simulink model "DrivetrainEv"  (R2023a)
settings: Solver=VariableStepAuto  StartTime=0.0  StopTime=inf  RelTol=1e-3  EnableMultiTasking=on
model workspace (MAT data in the model file):
  Af = Simulink.Parameter
  Af.Value = 2.27
  Af.DataType = 'double'
  Af.Complexity = 'real'
  Af.Dimensions = [1 1]
  Bx = Simulink.Parameter
  Bx.Value = 10
  Bx.DataType = 'double'
  Bx.Complexity = 'real'
  Bx.Dimensions = [1 1]
  Cd = Simulink.Parameter
  Cd.Value = 0.28
  Cd.DataType = 'double'
  Cd.Complexity = 'real'
  Cd.Dimensions = [1 1]
  Cl = Simulink.Parameter
  Cl.Value = 0.1
  Cl.DataType = 'double'
  Cl.Complexity = 'real'
  Cl.Dimensions = [1 1]
  Cpm = Simulink.Parameter
  Cpm.Value = 0.1
  Cpm.DataType = 'double'
  Cpm.Complexity = 'real'
  Cpm.Dimensions = [1 1]
  Cx = Simulink.Parameter
  Cx.Value = 1.65
  Cx.DataType = 'double'
  Cx.Complexity = 'real'
  Cx.Dimensions = [1 1]
  Dx = Simulink.Parameter
  Dx.Value = 1
  Dx.DataType = 'double'
  Dx.Complexity = 'real'
  Dx.Dimensions = [1 1]
  Ex = Simulink.Parameter
  Ex.Value = 0.01
  Ex.DataType = 'double'
  Ex.Complexity = 'real'
  Ex.Dimensions = [1 1]
  FZMAX = Simulink.Parameter
  FZMAX.Value = 6570
  FZMAX.DataType = 'double'
  FZMAX.Complexity = 'real'
  FZMAX.Dimensions = [1 1]
  FZMIN = Simulink.Parameter
  FZMIN.Value = 0
  FZMIN.DataType = 'double'
  FZMIN.Complexity = 'real'
  FZMIN.Dimensions = [1 1]
  Fc = Simulink.Parameter
  Fc.Value = 500
  Fc.DataType = 'double'
  Fc.Complexity = 'real'
  Fc.Dimensions = [1 1]
  FsbF = Simulink.Parameter
  FsbF.Value = [-700000 -7000 -700 0 700 7000 700000]
  FsbF.DataType = 'double'
  FsbF.Complexity = 'real'
  FsbF.Dimensions = [1 7]
  FsbR = Simulink.Parameter
  FsbR.Value = [-700000 -7000 -700 0 700 7000 700000]
  FsbR.DataType = 'double'
  FsbR.Complexity = 'real'
  FsbR.Dimensions = [1 7]
  FskF = Simulink.Parameter
  FskF.Value = [-8928.57142857 -178.571428571 0 357.142857143 535.714285714 9285.71428571]
  FskF.DataType = 'double'
  FskF.Complexity = 'real'
  FskF.Dimensions = [1 6]
  FskR = Simulink.Parameter
  FskR.Value = [-5357.14285714 -107.142857143 0 214.285714286 321.428571429 5571.42857143]
  FskR.DataType = 'double'
  FskR.Complexity = 'real'
  FskR.Dimensions = [1 6]
  Iyy = Simulink.Parameter
  Iyy.Value = 3000
  Iyy.DataType = 'double'
  Iyy.Complexity = 'real'
  Iyy.Dimensions = [1 1]
  Iyy_Whl = Simulink.Parameter
  Iyy_Whl.Value = 0.8
  Iyy_Whl.DataType = 'double'
  Iyy_Whl.Complexity = 'real'
  Iyy_Whl.Dimensions = [1 1]
  J = Simulink.Parameter
  J.Value = 0.01
  J.DataType = 'double'
  J.Complexity = 'real'
  J.Dimensions = [1 1]
  Jd = Simulink.Parameter
  Jd.Value = 0.025
  Jd.DataType = 'double'
  Jd.Complexity = 'real'
  Jd.Dimensions = [1 1]
  Jmotor = Simulink.Parameter
  Jmotor.Value = 0.1
  Jmotor.DataType = 'double'
  Jmotor.Complexity = 'real'
  Jmotor.Dimensions = [1 1]
  Jw1 = Simulink.Parameter
  Jw1.Value = 0.01
  Jw1.DataType = 'double'
  Jw1.Complexity = 'real'
  Jw1.Dimensions = [1 1]
  Jw2 = Simulink.Parameter
  Jw2.Value = 0.01
  Jw2.DataType = 'double'
  Jw2.Complexity = 'real'
  Jw2.Dimensions = [1 1]
  Lrel = Simulink.Parameter
  Lrel.Value = 0.15
  Lrel.DataType = 'double'
  Lrel.Complexity = 'real'
  Lrel.Dimensions = [1 1]
  Mass = Simulink.Parameter
  Mass.Value = 1500
  Mass.DataType = 'double'
  Mass.Complexity = 'real'
  Mass.Dimensions = [1 1]
  NF = Simulink.Parameter
  NF.Value = 2
  NF.DataType = 'double'
  NF.Complexity = 'real'
  NF.Dimensions = [1 1]
  NR = Simulink.Parameter
  NR.Value = 2
  NR.DataType = 'double'
  NR.Complexity = 'real'
  NR.Dimensions = [1 1]
  Ndiff = Simulink.Parameter
  Ndiff.Value = 7.94
  Ndiff.DataType = 'double'
  Ndiff.Complexity = 'real'
  Ndiff.Dimensions = [1 1]
  Ndisks = Simulink.Parameter
  Ndisks.Value = 4
  Ndisks.DataType = 'double'
  Ndisks.Complexity = 'real'
  Ndisks.Dimensions = [1 1]
  Pabs = Simulink.Parameter
  Pabs.Value = 101325
  Pabs.DataType = 'double'
  Pabs.Complexity = 'real'
  Pabs.Dimensions = [1 1]
  Re = Simulink.Parameter
  Re.Value = 0.327
  Re.DataType = 'double'
  Re.Complexity = 'real'
  Re.Dimensions = [1 1]
  Reff_LSD = Simulink.Parameter
  Reff_LSD.Value = 0.2
  Reff_LSD.DataType = 'double'
  Reff_LSD.Complexity = 'real'
  Reff_LSD.Dimensions = [1 1]
  Rm = Simulink.Parameter
  Rm.Value = 0.15
  Rm.DataType = 'double'
  Rm.Complexity = 'real'
  Rm.Dimensions = [1 1]
  T = Simulink.Parameter
  T.Value = 273
  T.DataType = 'double'
  T.Complexity = 'real'
  T.Dimensions = [1 1]
  UNLOADED_RADIUS = Simulink.Parameter
  UNLOADED_RADIUS.Value = 0.336
  UNLOADED_RADIUS.DataType = 'double'
  UNLOADED_RADIUS.Complexity = 'real'
  UNLOADED_RADIUS.Dimensions = [1 1]
  VXLOW = Simulink.Parameter
  VXLOW.Value = 2
  VXLOW.DataType = 'double'
  VXLOW.Complexity = 'real'
  VXLOW.Dimensions = [1 1]
  aMy = Simulink.Parameter
  aMy.Value = 0.01
  aMy.DataType = 'double'
  aMy.Complexity = 'real'
  aMy.Dimensions = [1 1]
  a_CG = Simulink.Parameter
  a_CG.Value = 1.188
  a_CG.DataType = 'double'
  a_CG.Complexity = 'real'
  a_CG.Dimensions = [1 1]
  alphaMy = Simulink.Parameter
  alphaMy.Value = 0
  alphaMy.DataType = 'double'
  alphaMy.Complexity = 'real'
  alphaMy.Dimensions = [1 1]
  b = Simulink.Parameter
  b.Value = 400
  b.DataType = 'auto'
  b.Complexity = 'real'
  b.Dimensions = [1 1]
  b1 = Simulink.Parameter
  b1.Value = 100
  b1.DataType = 'double'
  b1.Complexity = 'real'
  b1.Dimensions = [1 1]
  bMy = Simulink.Parameter
  bMy.Value = 0
  bMy.DataType = 'double'
  bMy.Complexity = 'real'
  bMy.Dimensions = [1 1]
  b_CG = Simulink.Parameter
  b_CG.Value = 1.512
  b_CG.DataType = 'double'
  b_CG.Complexity = 'real'
  b_CG.Dimensions = [1 1]
  b_J = Simulink.Parameter
  b_J.Value = 0.001
  b_J.DataType = 'double'
  b_J.Complexity = 'real'
  b_J.Dimensions = [1 1]
  bd = Simulink.Parameter
  bd.Value = 0.001
  bd.DataType = 'double'
  bd.Complexity = 'real'
  bd.Dimensions = [1 1]
  betaMy = Simulink.Parameter
  betaMy.Value = 1
  betaMy.DataType = 'double'
  betaMy.Complexity = 'real'
  betaMy.Dimensions = [1 1]
  br = Simulink.Parameter
  br.Value = 0.001
  br.DataType = 'double'
  br.Complexity = 'real'
  br.Dimensions = [1 1]
  bw1 = Simulink.Parameter
  bw1.Value = 0.001
  bw1.DataType = 'double'
  bw1.Complexity = 'real'
  bw1.Dimensions = [1 1]
  bw2 = Simulink.Parameter
  bw2.Value = 0.001
  bw2.DataType = 'double'
  bw2.Complexity = 'real'
  bw2.Dimensions = [1 1]
  cMy = Simulink.Parameter
  cMy.Value = 0
  cMy.DataType = 'double'
  cMy.Complexity = 'real'
  cMy.Dimensions = [1 1]
  disk_abore = Simulink.Parameter
  disk_abore.Value = 0.05
  disk_abore.DataType = 'double'
  disk_abore.Complexity = 'real'
  disk_abore.Dimensions = [1 1]
  domega_o = Simulink.Parameter
  domega_o.Value = 0
  domega_o.DataType = 'double'
  domega_o.Complexity = 'real'
  domega_o.Dimensions = [1 1]
  dw = Simulink.Parameter
  dw.Value = [0 10 20 40 60 80 100]
  dw.DataType = 'double'
  dw.Complexity = 'real'
  dw.Dimensions = [1 7]
  dzdotsF = Simulink.Parameter
  dzdotsF.Value = [-10 -1 -0.1 0 0.1 1 10]
  dzdotsF.DataType = 'double'
  dzdotsF.Complexity = 'real'
  dzdotsF.Dimensions = [1 7]
  dzdotsR = Simulink.Parameter
  dzdotsR.Value = [-10 -1 -0.1 0 0.1 1 10]
  dzdotsR.DataType = 'double'
  dzdotsR.Complexity = 'real'
  dzdotsR.Dimensions = [1 7]
  dzsF = Simulink.Parameter
  dzsF.Value = [-0.005 -0.0001 0 0.2 0.2001 0.2051]
  dzsF.DataType = 'double'
  dzsF.Complexity = 'real'
  dzsF.Dimensions = [1 6]
  dzsR = Simulink.Parameter
  dzsR.Value = [-0.005 -0.0001 0 0.2 0.2001 0.2051]
  dzsR.DataType = 'double'
  dzsR.Complexity = 'real'
  dzsR.Dimensions = [1 6]
  g = Simulink.Parameter
  g.Value = 9.81
  g.DataType = 'double'
  g.Complexity = 'real'
  g.Dimensions = [1 1]
  h = Simulink.Parameter
  h.Value = 0.5
  h.DataType = 'double'
  h.Complexity = 'real'
  h.Dimensions = [1 1]
  k = Simulink.Parameter
  k.Value = 10000
  k.DataType = 'auto'
  k.Complexity = 'real'
  k.Dimensions = [1 1]
  k1 = Simulink.Parameter
  k1.Value = 50000
  k1.DataType = 'double'
  k1.Complexity = 'real'
  k1.Dimensions = [1 1]
  kappamax = Simulink.Parameter
  kappamax.Value = 1.5
  kappamax.DataType = 'double'
  kappamax.Complexity = 'real'
  kappamax.Dimensions = [1 1]
  lam_x = Simulink.Parameter
  lam_x.Value = 1
  lam_x.DataType = 'double'
  lam_x.Complexity = 'real'
  lam_x.Dimensions = [1 1]
  mu_kinetic = Simulink.Parameter
  mu_kinetic.Value = 0.35
  mu_kinetic.DataType = 'double'
  mu_kinetic.Complexity = 'real'
  mu_kinetic.Dimensions = [1 1]
  mu_static = Simulink.Parameter
  mu_static.Value = 0.45
  mu_static.DataType = 'double'
  mu_static.Complexity = 'real'
  mu_static.Dimensions = [1 1]
  muc = Simulink.Parameter
  muc.Value = [0.16 0.13 0.115 0.11 0.105 0.1025 0.10125]
  muc.DataType = 'double'
  muc.Complexity = 'real'
  muc.Dimensions = [1 7]
  num_pads = Simulink.Parameter
  num_pads.Value = 2
  num_pads.DataType = 'double'
  num_pads.Complexity = 'real'
  num_pads.Dimensions = [1 1]
  omega1_c = Simulink.Parameter
  omega1_c.Value = 3000
  omega1_c.DataType = 'double'
  omega1_c.Complexity = 'real'
  omega1_c.Dimensions = [1 1]
  omega_c = Simulink.Parameter
  omega_c.Value = 100
  omega_c.DataType = 'auto'
  omega_c.Complexity = 'real'
  omega_c.Dimensions = [1 1]
  omega_o = Simulink.Parameter
  omega_o.Value = 0
  omega_o.DataType = 'double'
  omega_o.Complexity = 'real'
  omega_o.Dimensions = [1 1]
  omega_o_J = Simulink.Parameter
  omega_o_J.Value = 0
  omega_o_J.DataType = 'double'
  omega_o_J.Complexity = 'real'
  omega_o_J.Dimensions = [1 1]
  omegao = Simulink.Parameter
  omegao.Value = 0
  omegao.DataType = 'double'
  omegao.Complexity = 'real'
  omegao.Dimensions = [1 1]
  omegaw1o = Simulink.Parameter
  omegaw1o.Value = 0
  omegaw1o.DataType = 'double'
  omegaw1o.Complexity = 'real'
  omegaw1o.Dimensions = [1 1]
  omegaw2o = Simulink.Parameter
  omegaw2o.Value = 0
  omegaw2o.DataType = 'double'
  omegaw2o.Complexity = 'real'
  omegaw2o.Dimensions = [1 1]
  press = Simulink.Parameter
  press.Value = 234400
  press.DataType = 'double'
  press.Complexity = 'real'
  press.Dimensions = [1 1]
  q_o = Simulink.Parameter
  q_o.Value = 0
  q_o.DataType = 'double'
  q_o.Complexity = 'real'
  q_o.Dimensions = [1 1]
  tauC_LSD = Simulink.Parameter
  tauC_LSD.Value = 0.01
  tauC_LSD.DataType = 'double'
  tauC_LSD.Complexity = 'real'
  tauC_LSD.Dimensions = [1 1]
  theta_o = Simulink.Parameter
  theta_o.Value = 0
  theta_o.DataType = 'double'
  theta_o.Complexity = 'real'
  theta_o.Dimensions = [1 1]
  theta_o_Veh = Simulink.Parameter
  theta_o_Veh.Value = 0
  theta_o_Veh.DataType = 'double'
  theta_o_Veh.Complexity = 'real'
  theta_o_Veh.Dimensions = [1 1]
  wc_shaft = Simulink.Parameter
  wc_shaft.Value = 0.1
  wc_shaft.DataType = 'auto'
  wc_shaft.Complexity = 'real'
  wc_shaft.Dimensions = [1 1]
  x_o = Simulink.Parameter
  x_o.Value = 0
  x_o.DataType = 'double'
  x_o.Complexity = 'real'
  x_o.Dimensions = [1 1]
  xdot_o = Simulink.Parameter
  xdot_o.Value = 0
  xdot_o.DataType = 'double'
  xdot_o.Complexity = 'real'
  xdot_o.Dimensions = [1 1]
  z_o = Simulink.Parameter
  z_o.Value = -0.35
  z_o.DataType = 'double'
  z_o.Complexity = 'real'
  z_o.Dimensions = [1 1]
  zdot_o = Simulink.Parameter
  zdot_o.Value = 0
  zdot_o.DataType = 'double'
  zdot_o.Complexity = 'real'
  zdot_o.Dimensions = [1 1]
libraries: autolibsharedcoupling x8, autolibpowerinfoutils x6, autolibshareddiff x4, autolibshared x3
(part 1 of 3)
settings Model: DataDictionary=DrivetrainEv.sldd  ModifiedByFormat=The MathWorks, Inc.  SimulationMode=accelerator  PauseTimes=10  Creator=The MathWorks, Inc.  LastModifiedBy=The MathWorks, Inc.
settings SolverCC: AlgebraicLoopSolver=TrustRegion  DecoupledContinuousIntegration=on  MinimalZcImpactIntegration=on  MaxZcPerStep=1
settings DataIOCC: DSMLogging=off  ReturnWorkspaceOutputs=off
settings DebuggingCC: MergeDetectMultiDrivingBlocksExec=none  UnconnectedInputMsg=warning  UnconnectedOutputMsg=warning  UnconnectedLineMsg=warning  PregeneratedLibrarySubsystemCodeDiagnostic=none  ArithmeticOperatorsInVariantConditions=warning
settings ModelReferenceCC: EnableRefExpFcnMdlSchedulingChecks=on  PropagateSignalLabelsOutOfModel=off
settings SFSimCC: SimUseLocalCustomCode=off
settings RTWCC: RTWUseLocalCustomCode=off  DLArmComputeVersion=19.05
settings CodeAppCC: StateflowObjectComments=on
settings GRTTargetCC: TargetLangStandard=C89/C90 (ANSI)
settings ConfigComp: CovMetricSettings=dsw  CovSaveCumulativeToWorkspaceVar=on  CovSaveSingleToWorkspaceVar=on  CovExternalEMLEnable=off
settings SimscapeCC: SimscapeNormalizeSystem=off

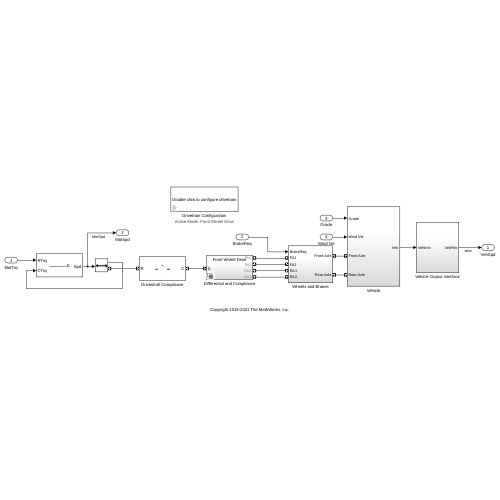
[thumbnail: Simulink's stored preview of the top-level diagram]
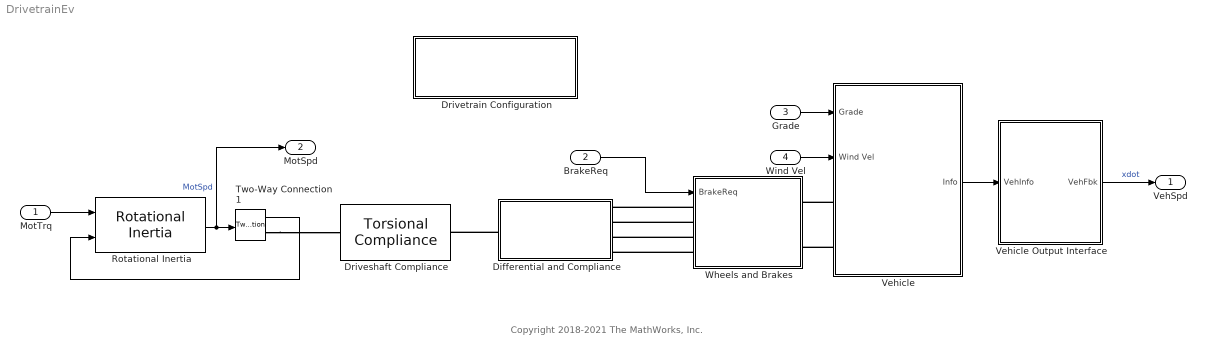
== system DrivetrainEv ==
  note: Copyright 2018-2021 The MathWorks, Inc.
  MotTrq : Inport
  BrakeReq : Inport  Port=2
  Grade : Inport  Port=3
  Wind Vel : Inport  Port=4
  Differential and Compliance : Subsystem  Variant=on  VariantControlMode=label  LabelModeActiveChoice=0
  Driveshaft Compliance : autolibsharedcoupling/Torsional Compliance  port_config=Two-way connection  extInfo=off  k=k  b=b  theta_o=theta_o  domega_o=domega_o  omega_c=omega_c  blkID=0  aMode=1
  Drivetrain Configuration : Subsystem  mask(Drivetrain Configuration){drivetrainMode=Front Wheel Drive}
      mask prompts: drivetrainMode "Drivetrain Mode"
      mask help: Use this block to configure the dirvetrain mode.
      settings: AttributesFormatString=Active Mode: %<drivetrainMode>
      mask TypeOptions drivetrainMode: Front Wheel Drive | Rear Wheel Drive | All Wheel Drive
      mask Callback drivetrainMode:
      | switch get_param(gcb,'drivetrainMode')
      |     case 'Front Wheel Drive'
      |         set_param([bdroot '/Differential and Compliance'],'OverrideUsingVariant','0')
      |     case 'Rear Wheel Drive'
      |         set_param([bdroot '/Differential and Compliance'],'OverrideUsingVariant','1')
      |     case 'All Wheel Drive'
      |         set_param([bdroot '/Differential and Compliance'],'OverrideUsingVariant','2')
      |     otherwise
      |         set_param([bdroot '/Differential and Compliance'],'OverrideUsingVariant','0')
      | end
      mask Display: disp('Double click to configure drivetrain')
  Rotational Inertia : autolibsharedcoupling/Rotational Inertia  port_config=Simulink  extInfo=off  externJ=off  J=Jmotor  b=.001  omega_o=omega_o  blkID=0  aMode=1
      settings: LibrarySourceBlock=autolibcoupling/Rotational Inertia
  Two-Way Connection1 : TwoWayConnection
  Vehicle : Subsystem
  Vehicle Output Interface : Subsystem
  Wheels and Brakes : Subsystem  VariantControl=0
  VehSpd : Outport  VectorParamsAs1DForOutWhenUnconnected=off
  MotSpd : Outport  Port=2  VectorParamsAs1DForOutWhenUnconnected=off  BusOutputAsStruct=on
  wires:
  BrakeReq/1 -> Wheels and Brakes/1(BrakeReq)
  Vehicle/1(Info) -> Vehicle Output Interface/1(VehInfo)
  Vehicle Output Interface/1(VehFbk) -> VehSpd/1  "xdot"
  Rotational Inertia/1 -> MotSpd/1, Two-Way Connection1/1  "MotSpd"
  Wind Vel/1 -> Vehicle/2(Wind Vel)
  Grade/1 -> Vehicle/1(Grade)
  MotTrq/1 -> Rotational Inertia/1
  Two-Way Connection1/1 -> Rotational Inertia/2
  connections:
  Differential and Compliance/LConn1 -- Driveshaft Compliance/RConn1
  Wheels and Brakes/LConn1 -- Differential and Compliance/RConn1
  Wheels and Brakes/LConn2 -- Differential and Compliance/RConn2
  Wheels and Brakes/LConn3 -- Differential and Compliance/RConn3
  Wheels and Brakes/LConn4 -- Differential and Compliance/RConn4
  Vehicle/LConn1 -- Wheels and Brakes/RConn1
  Vehicle/LConn2 -- Wheels and Brakes/RConn2
  Two-Way Connection1/RConn1 -- Driveshaft Compliance/LConn1

== system DrivetrainEv/Differential and Compliance ==
  All Wheel Drive : Subsystem  VariantControl=2
  Front Wheel Drive : Subsystem  VariantControl=0
  Rear Wheel Drive : Subsystem  VariantControl=1
  D : PMIOPort  Side=Left
  FA1 : PMIOPort  Port=2  Side=Right
  FA2 : PMIOPort  Port=3  Side=Right
  RA1 : PMIOPort  Port=4  Side=Right
  RA2 : PMIOPort  Port=5  Side=Right

== system DrivetrainEv/Drivetrain Configuration ==

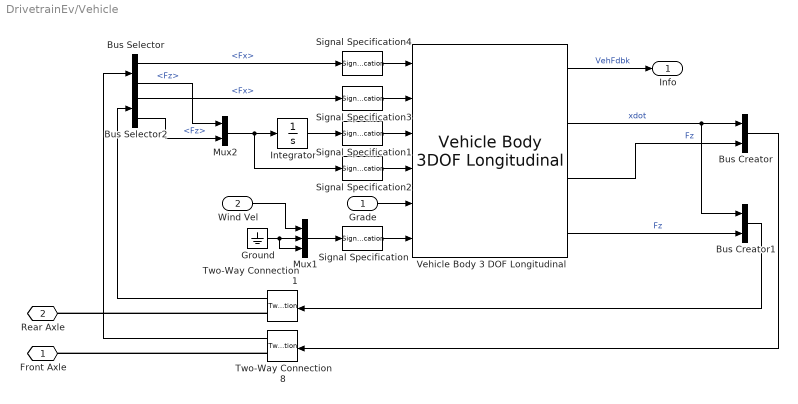
== system DrivetrainEv/Vehicle ==
  Grade : Inport  Unit=deg
  Wind Vel : Inport  Port=2  Unit=m/s
  Bus Creator : BusCreator  Inputs=2
  Bus Creator1 : BusCreator  Inputs=2
  Bus Selector : BusSelector  OutputSignals=Fx,Fz
  Bus Selector2 : BusSelector  OutputSignals=Fx,Fz
  Ground : Ground
  Integrator : Integrator
  Mux1 : Mux  Inputs=3
  Mux2 : Mux  Inputs=2
  Signal Specification : SignalSpecification  Unit=m/s
  Signal Specification1 : SignalSpecification  Unit=m
  Signal Specification2 : SignalSpecification  Unit=m/s
  Signal Specification3 : SignalSpecification  Unit=N
  Signal Specification4 : SignalSpecification  Unit=N
  Two-Way Connection1 : TwoWayConnection
  Two-Way Connection8 : TwoWayConnection
  Vehicle Body 3 DOF Longitudinal : autolibshared/Vehicle Body 3DOF Longitudinal  VariantControl=SL  groundType=Axle displacement, velocity  aMode=1  extFMode=off  extMMode=off  extTamb=off  NF=NF  NR=NR  m=Mass  a=a_CG  b=b_CG  h=h  Cd=Cd  Af=Af  x_o=x_o  xdot_o=xdot_o  Cl=Cl  z_o=z_o  zdot_o=zdot_o  Iyy=Iyy  Cpm=Cpm  theta_o=theta_o_Veh  q_o=q_o  FskF=FskF  dzsF=dzsF  FsbF=FsbF  dzdotsF=dzdotsF  FskR=FskR  dzsR=dzsR  FsbR=FsbR  dzdotsR=dzdotsR  Pabs=Pabs  T=T  g=g  blkID=0
      settings: LibrarySourceBlock=autolibvehdynlong/Vehicle Body 3DOF Longitudinal
  Front Axle : PMIOPort  Side=Left
  Rear Axle : PMIOPort  Port=2  Side=Left
  Info : Outport  VectorParamsAs1DForOutWhenUnconnected=off
  wires:
  Two-Way Connection1/1 -> Bus Selector2/1
  Bus Selector2/2 -> Mux2/2  "<Fz>"
  Bus Selector2/1 -> Signal Specification3/1  "<Fx>"
  Bus Selector/2 -> Mux2/1  "<Fz>"
  Bus Selector/1 -> Signal Specification4/1  "<Fx>"
  Bus Creator1/1 -> Two-Way Connection1/1
  Bus Creator/1 -> Two-Way Connection8/1
  Signal Specification4/1 -> Vehicle Body 3 DOF Longitudinal/1
  Signal Specification3/1 -> Vehicle Body 3 DOF Longitudinal/2
  Signal Specification2/1 -> Vehicle Body 3 DOF Longitudinal/4
  Signal Specification1/1 -> Vehicle Body 3 DOF Longitudinal/3
  Signal Specification/1 -> Vehicle Body 3 DOF Longitudinal/6
  Grade/1 -> Vehicle Body 3 DOF Longitudinal/5
  Wind Vel/1 -> Mux1/1
  Integrator/1 -> Signal Specification1/1
  Mux2/1 -> Signal Specification2/1, Integrator/1
  Vehicle Body 3 DOF Longitudinal/4 -> Bus Creator1/2  "Fz"
  Mux1/1 -> Signal Specification/1
  Ground/1 -> Mux1/3, Mux1/2
  Vehicle Body 3 DOF Longitudinal/1 -> Info/1  "VehFdbk"
  Two-Way Connection8/1 -> Bus Selector/1
  Vehicle Body 3 DOF Longitudinal/2 -> Bus Creator/1, Bus Creator1/1  "xdot"
  Vehicle Body 3 DOF Longitudinal/3 -> Bus Creator/2  "Fz"
  connections:
  Two-Way Connection1/RConn1 -- Rear Axle/RConn1
  Two-Way Connection8/RConn1 -- Front Axle/RConn1

== system DrivetrainEv/Vehicle Output Interface ==
  VehInfo : Inport
  Bus Selector1 : BusSelector  OutputSignals=BdyFrm.Cg.Vel.xdot
  VehFbk : Outport  VectorParamsAs1DForOutWhenUnconnected=off
  wires:
  Bus Selector1/1 -> VehFbk/1  "<xdot>"
  VehInfo/1 -> Bus Selector1/1
